simulink model "q1"  (R2021a)
settings: Solver=VariableStepAuto  StartTime=0.0  StopTime=10.0  RelTol=1e-3
settings Model: Creator=louis  LastModifiedBy=louis
settings DataIOCC: ExternalInput=untitledScenario.getElement('In1')  LoadExternalInput=on

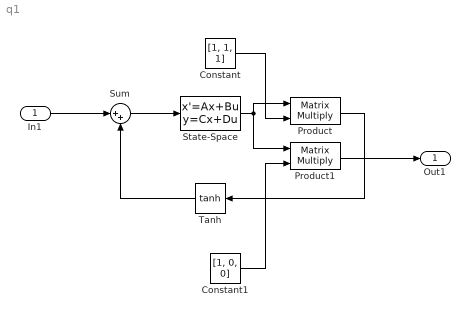
== system q1 ==
  In1 : Inport  PortDimensions=1
  Constant : Constant  Value=[1, 1, 1]
  Constant1 : Constant  Value=[1, 0, 0]
  Product : Product  Multiplication=Matrix(*)
  Product1 : Product  Multiplication=Matrix(*)
  State-Space : StateSpace  A=[-10, 0, 10; 0, -100, 100; 0, 0, -1]  B=[0; 0; 1]  C=eye(3)  D=zeros(3,1)  InitialCondition=0
  Sum : Sum  Inputs=|++
  Tanh : Trigonometry  Operator=tanh
  Out1 : Outport  PortDimensions=1
  wires:
  Sum/1 -> State-Space/1
  In1/1 -> Sum/1
  Tanh/1 -> Sum/2
  Product/1 -> Tanh/1
  Constant1/1 -> Product1/2
  Product1/1 -> Out1/1
  Constant/1 -> Product/2
  State-Space/1 -> Product1/1, Product/1
